simulink model "pwm_ppm_self"  (R2018a)
settings: Solver=VariableStepAuto  StartTime=0.0  StopTime=10  RelTol=1e-3
libraries: powerlib_meascontrol x3, dsparch4 x2, simulink x1
settings Model: Creator=hp  LastModifiedBy=hp

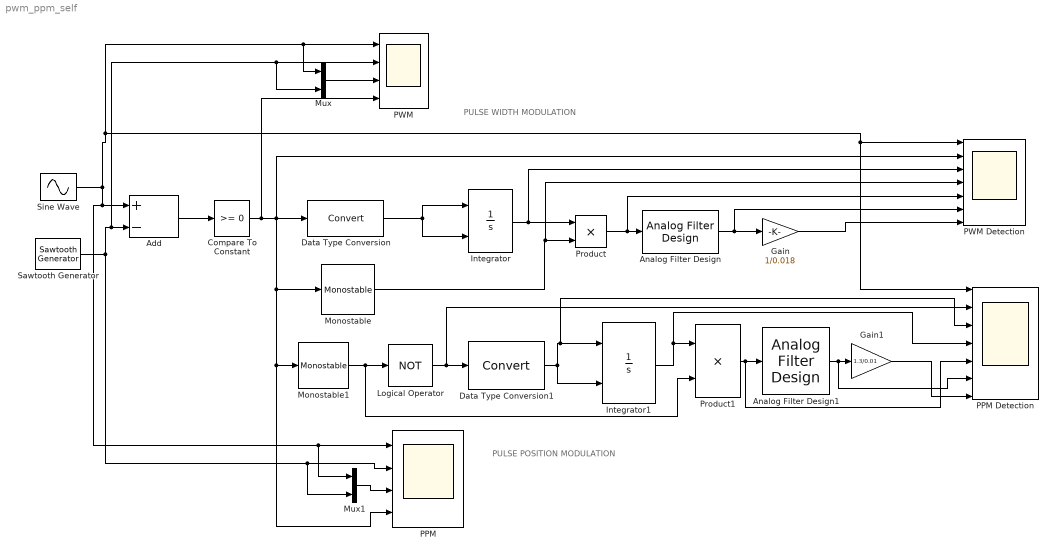
== system pwm_ppm_self ==
  note: PULSE POSITION MODULATION
  note: PULSE WIDTH MODULATION
  Add : Sum  Inputs=+-
  Analog Filter Design : dsparch4/Analog Filter Design  method=Chebyshev I  filttype=Bandpass  N=2  Wlo=2*pi*1.5  Whi=2*pi*2.5  Rp=2  Rs=40
  Analog Filter Design1 : dsparch4/Analog Filter Design  method=Chebyshev I  filttype=Bandpass  N=2  Wlo=2*pi*1.5  Whi=2*pi*2.5  Rp=2  Rs=40
  Compare To Constant : simulink/Logic and Bit Operations/Compare To Constant  relop=>=  const=0  OutDataTypeStr=boolean
  Data Type Conversion : DataTypeConversion
  Data Type Conversion1 : DataTypeConversion
  Gain : Gain  Gain=1/0.018
  Gain1 : Gain  Gain=1.3/0.01
  Integrator : Integrator  ExternalReset=rising
  Integrator1 : Integrator  ExternalReset=rising
  Logical Operator : Logic  Operator=NOT  Inputs=1  AllPortsSameDT=off  OutDataTypeStr=boolean
  Monostable : powerlib_meascontrol/Logic/Monostable  EdgeDetect=Falling  PulseDuration=0.05  ic=0  Ts=0
      settings: SourceProductName=Simscape Power Systems  SourceProductBaseCode=PS
  Monostable1 : powerlib_meascontrol/Logic/Monostable  EdgeDetect=Falling  PulseDuration=0.015  ic=0  Ts=0
      settings: SourceProductName=Simscape Power Systems  SourceProductBaseCode=PS
  Mux : Mux  Inputs=2
  Mux1 : Mux  Inputs=2
  PPM : Scope  NumInputPorts=4
  PPM Detection : Scope  NumInputPorts=7
  PWM : Scope  NumInputPorts=4
  PWM Detection : Scope  NumInputPorts=7
  Product : Product
  Product1 : Product
  Sawtooth Generator : powerlib_meascontrol/Pulse & Signal Generators/Sawtooth Generator  Freq=10  Phase=0  Ts=0
      settings: SourceProductName=Simscape Power Systems
  Sine Wave : Sin  Frequency=2*pi*2  SampleTime=0
  wires:
  Add/1 -> Compare To Constant/1
  Compare To Constant/1 -> PWM/4, PWM Detection/2, PPM/4, Monostable1/1, Monostable/1, Data Type Conversion/1
  Data Type Conversion/1 -> Integrator/2, Integrator/1
  Integrator/1 -> PWM Detection/3, Product/1
  Monostable/1 -> PWM Detection/4, Product/2
  Product/1 -> PWM Detection/5, Analog Filter Design/1
  Gain/1 -> PWM Detection/7
  Sine Wave/1 -> Mux/1, PWM/1, PPM Detection/1, PWM Detection/1, Mux1/1, PPM/1, Add/1
  Analog Filter Design/1 -> PWM Detection/6, Gain/1
  Sawtooth Generator/1 -> Mux1/2, PPM/2, Mux/2, PWM/2, Add/2
  Monostable1/1 -> Product1/2, Logical Operator/1
  Logical Operator/1 -> PPM Detection/2, Data Type Conversion1/1
  Data Type Conversion1/1 -> Integrator1/2, PPM Detection/3, Integrator1/1
  Integrator1/1 -> PPM Detection/4, Product1/1
  Product1/1 -> PPM Detection/5, Analog Filter Design1/1
  Analog Filter Design1/1 -> PPM Detection/6, Gain1/1
  Gain1/1 -> PPM Detection/7
  Mux/1 -> PWM/3
  Mux1/1 -> PPM/3
